simulink library "BandSplitLib"  (R2022b)
settings: Solver=VariableStepAuto  StartTime=0.0  StopTime=10.0  RelTol=1e-3
libraries: FeaturePath x1, FirDown x1, FirUp x1, HandyTextFile x1
settings Model: Creator=jb1046154  LastModifiedBy=fz1054048
settings SolverCC: AlgebraicLoopSolver=TrustRegion
settings DebuggingCC: UnconnectedInputMsg=warning  UnconnectedOutputMsg=warning  UnconnectedLineMsg=warning  SFMachineParentedDataDiag=warning
settings ModelReferenceCC: EnableRefExpFcnMdlSchedulingChecks=on

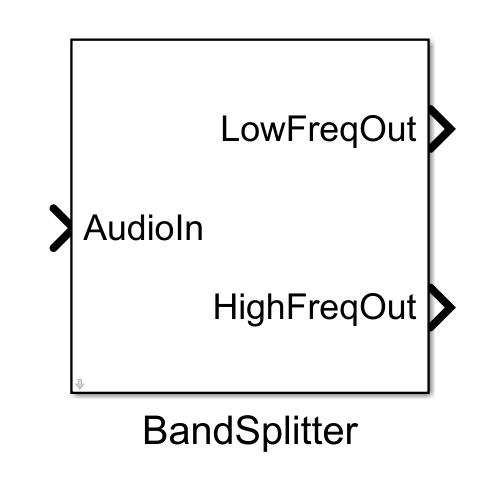
[thumbnail: Simulink's stored preview of the top-level diagram]
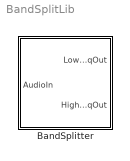
== system BandSplitLib ==
  BandSplitter : Subsystem  mask(Blocklib BandSplitter){Config=[], FeatureName=BandSplit}
      mask prompts: Config "BandSplitterConfig"; FeatureName "Feature path name:"
      mask help:
      | See help for more information
      | or run
      | >> help BandSplitterConfig
      mask init:
      | blkh=gcbh;
      | Config=BTConfig.Assert(blkh,Config);
      | 
      | Config.Validate();
      | Config.DoMaskInit(blkh);
      mask Help: eval('help BandSplitterConfig')
      mask TypeOptions FeatureName: FeaturePath/FeatureName

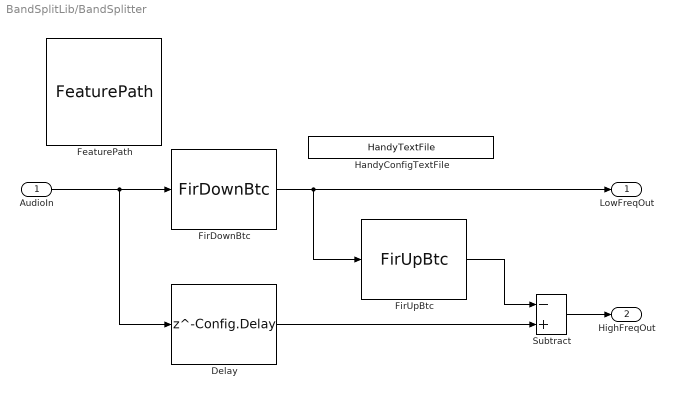
== system BandSplitLib/BandSplitter ==
  AudioIn : Inport
  Delay : Delay  DelayLength=Config.Delay  InitialCondition=0  InputProcessing=Columns as channels (frame based)  UseCircularBuffer=on
  FeaturePath : FeaturePath/FeaturePath  FeatureName=BandSplit  IsGroup=off  GroupNumber=-1  IsModule=off  TriggerInit=[-165 -26 -50 81]
      settings: SourceProductName=Bose Talaria
  FirDownBtc : FirDown/FirDownBtc  Config=Config.FirDown  FeatureName=FirDown
      settings: SourceProductName=Bose Blocklib
  FirUpBtc : FirUp/FirUpBtc  Config=Config.FirUp  FeatureName=FirUp
      settings: SourceProductName=Bose Blocklib
  HandyConfigTextFile : HandyTextFile/HandyTextFile  TemplateSource=Config  FileSuffix=File  OpenDialogOnLoad=off  UseThisBlockName=off  AddGrandParentNamePrefix=off  TheDefaultText=% $(FILENAME) $(PREFIX) $(SUFFIX)  ShowInLibBrowser=on
      settings: SourceProductName=Bose Talaria
  Subtract : Sum  Inputs=-+
  LowFreqOut : Outport
  HighFreqOut : Outport  Port=2
  wires:
  AudioIn/1 -> Delay/1, FirDownBtc/1
  FirDownBtc/1 -> LowFreqOut/1, FirUpBtc/1
  FirUpBtc/1 -> Subtract/1
  Delay/1 -> Subtract/2
  Subtract/1 -> HighFreqOut/1
